simulink model "Vehicle1D_harness_model"  (R2021a)
settings: Solver=daessc  StartTime=0.0  StopTime=t_end  RelTol=1e-3  AbsTol=1e-3
PreLoadFcn:
  | Vehicle1D_harness_setup
undefined symbols (not defined in the file): gearTrain
libraries: fl_lib x5, nesl_utility x2
settings Model: Creator=isaacito  LastModifiedBy=isaacito
settings SolverCC: AutoScaleAbsTol=off  AlgebraicLoopSolver=TrustRegion
settings DebuggingCC: SFMachineParentedDataDiag=warning
settings SimscapeCC: SimscapeLogType=all  SimscapeLogSimulationStatistics=on  SimscapeLogLimitData=off

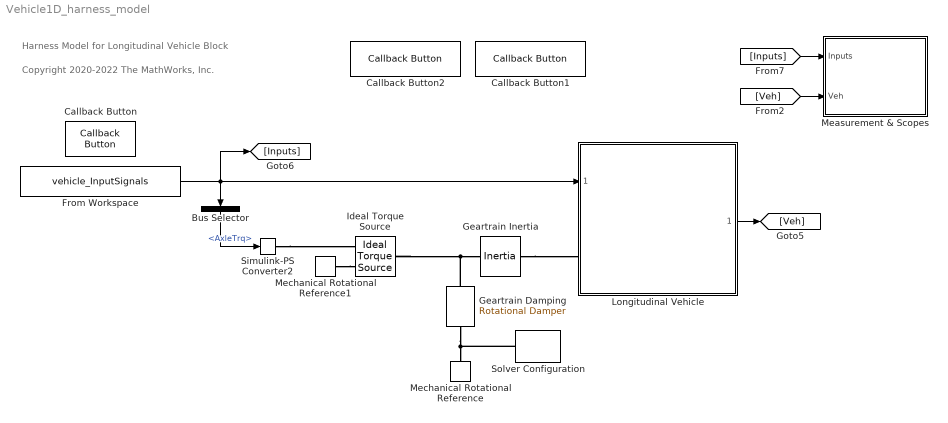
== system Vehicle1D_harness_model ==
  note: Harness Model for Longitudinal Vehicle Block
  note: Copyright 2020-2022 The MathWorks, Inc.
  Bus Selector : BusSelector  OutputSignals=AxleTrq
  Callback Button : CallbackButton  ButtonText=Plot input
      settings: ClickFcn="Vehicle1D_plot_inputs(\"vehicle_InputSignals\")"
  Callback Button1 : CallbackButton  ButtonText=Open Set-Up Script
      settings: ClickFcn=edit Vehicle1D_harness_setup
  Callback Button2 : CallbackButton  ButtonText=Open Main Script
      settings: ClickFcn=edit Vehicle1D_main_script
  From Workspace : FromWorkspace  VariableName=vehicle_InputSignals  OutDataTypeStr=Bus: vehicle_InputBus  Interpolate=off  OutputAfterFinalValue=Holding final value
      settings: AttributesFormatString=|
      | %<OutDataTypeStr>
      | Interpolate: %<Interpolate>
  Geartrain Damping : fl_lib/Mechanical/Rotational Elements/Rotational Damper  D=gearTrain.friction_Nm_per_rpm m*N/rpm  w_specify=off  w_priority=None  w=0 rad/s  w_nominal_specify=off  w_nominal_unit=rad/s  w_nominal_value=1  t_specify=off  t_priority=None  t=0 N*m  t_nominal_specify=off  t_nominal_unit=N*m  t_nominal_value=1
      settings: AttributesFormatString=|
      | %<D>
      | %<D_unit>
  Geartrain Inertia : fl_lib/Mechanical/Rotational Elements/Inertia  inertia=gearTrain.inertia_kg_m2 kg*m^2  num_ports=foundation.enum.numPorts2.two  w_specify=on  w_priority=None  w=0 rpm  w_nominal_specify=off  w_nominal_unit=rad/s  w_nominal_value=1  t_specify=off  t_priority=None  t=0 N*m  t_nominal_specify=off  t_nominal_unit=N*m  t_nominal_value=1
      settings: InternalSimscapePortConfiguration="{\"Bottom\":[],\"Left\":[{\"id\":\"I\",\"label\":\"\",\"type\":\"foundation.mechanical.rotational.rotational\"}],\"Right\":[{\"id\":\"J\",\"label\":\"\",\"type\":\"foundation.mechanical.rotational.rotational\"}],\"Top\":[]}"
      settings: AttributesFormatString=|
      | %<inertia>
      | %<inertia_unit>
  Ideal Torque Source : fl_lib/Mechanical/Mechanical Sources/Ideal Torque Source
  Longitudinal Vehicle : Subsystem  ReferencedSubsystem=Vehicle1DCustom_refsub
  Measurement & Scopes : Subsystem
  Mechanical Rotational Reference : fl_lib/Mechanical/Rotational Elements/Mechanical Rotational Reference
  Mechanical Rotational Reference1 : fl_lib/Mechanical/Rotational Elements/Mechanical Rotational Reference
  Simulink-PS Converter2 : nesl_utility/Simulink-PS Converter  PhysicalDomain=network_engine_domain  SubClassName=ps_input  LeftPortType=input  RightPortType=output  PseudoPeriodic=off  Frequencies=[]  NoiseDistribution=none  NoiseParameters=[]  Unit=N*m  AffineConversion=off  FilteringAndDerivatives=filter  SimscapeFilterOrder=1  InputFilterTimeConstant=0.001  UdotUserProvided=0
      settings: SourceProductBaseCode=PW,SS
  Solver Configuration : nesl_utility/Solver Configuration  PhysicalDomain=network_engine_domain  SubClassName=solver  LeftPortType=input  RightPortType=generic  Tones=[]  Harmonics=[]  SimulateNoise=off  Profile=off  UseLocalSampling=off  EnableSwitchedLinearOptims=on  FrequencyDomain=off  UseCCode=off  RelTol=0.001  AbsTol=1e-06  MinStep=1e-09  ToWorkspace=off  RevertToSquareIcSolve=off  NumHomotopyIterations=100  PhasorMode=off  PhasorModeNumHarmonics=1  DoDC=off  ResidualTolerance=1e-09  UseLocalSolver=off  LocalSolverChoice=NE_BACKWARD_EULER_ADVANCER  LocalSolverSampleTime=0.001  DoFixedCost=off  MaxNonlinIter=3  MaxModeIter=2  ComputeImpulses=off  ImpulseIterations=2  LinearAlgebra=auto  EquationFormulation=NE_TIME_EF  DelaysMemoryBudget=1024  AutomaticFiltering=on  FilteringTimeConstant=0.001  PartitionStorageMethod=AS_NEEDED  PartitionMemoryBudget=1024  PartitionMethod=ROBUST
      settings: AttributesFormatString=Local solver %<UseLocalSolver>  SourceProductBaseCode=PW,SS
  wires:
  Longitudinal Vehicle/1 -> [Veh]
  Bus Selector/1 -> Simulink-PS Converter2/1  "<AxleTrq>"
  From Workspace/1 -> [Inputs], Longitudinal Vehicle/1, Bus Selector/1
  [Veh] -> Measurement & Scopes/2(Veh)
  [Inputs] -> Measurement & Scopes/1(Inputs)
  connections:
  Geartrain Damping/RConn1 -- Solver Configuration/RConn1 -- Mechanical Rotational Reference/LConn1
  Simulink-PS Converter2/RConn1 -- Ideal Torque Source/RConn1
  Mechanical Rotational Reference1/LConn1 -- Ideal Torque Source/RConn2
  Geartrain Inertia/LConn1 -- Longitudinal Vehicle/LConn1
  Ideal Torque Source/LConn1 -- Geartrain Damping/LConn1 -- Geartrain Inertia/RConn1

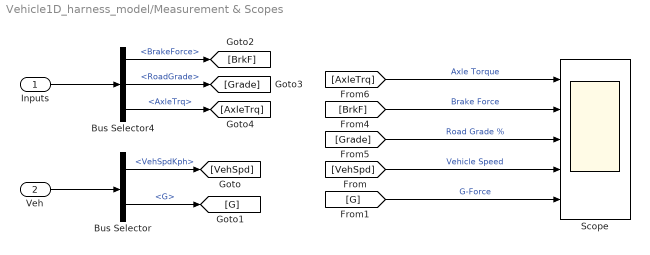
== system Vehicle1D_harness_model/Measurement & Scopes ==
  Inputs : Inport
  Veh : Inport  Port=2
  Bus Selector : BusSelector  OutputSignals=VehSpdKph,G
  Bus Selector4 : BusSelector  OutputSignals=BrakeForce,RoadGrade,AxleTrq
  Scope : Scope  NumInputPorts=5
  wires:
  Bus Selector4/2 -> [Grade]  "<RoadGrade>"
  [VehSpd] -> Scope/4  "Vehicle Speed"
  [G] -> Scope/5  "G-Force"
  [AxleTrq] -> Scope/1  "Axle Torque"
  Bus Selector4/3 -> [AxleTrq]  "<AxleTrq>"
  Bus Selector4/1 -> [BrkF]  "<BrakeForce>"
  Inputs/1 -> Bus Selector4/1
  Bus Selector/2 -> [G]  "<G>"
  Veh/1 -> Bus Selector/1
  Bus Selector/1 -> [VehSpd]  "<VehSpdKph>"
  [Grade] -> Scope/3  "Road Grade %"
  [BrkF] -> Scope/2  "Brake Force"
